simulink model "simulation"  (R2018b)
settings: Solver=ode45  StartTime=0.0  StopTime=36  FixedStep=0.00001  MaxStep=0.00001  MinStep=0.000005  RelTol=1e-3
settings Model: Creator=Dell  LastModifiedBy=Dell

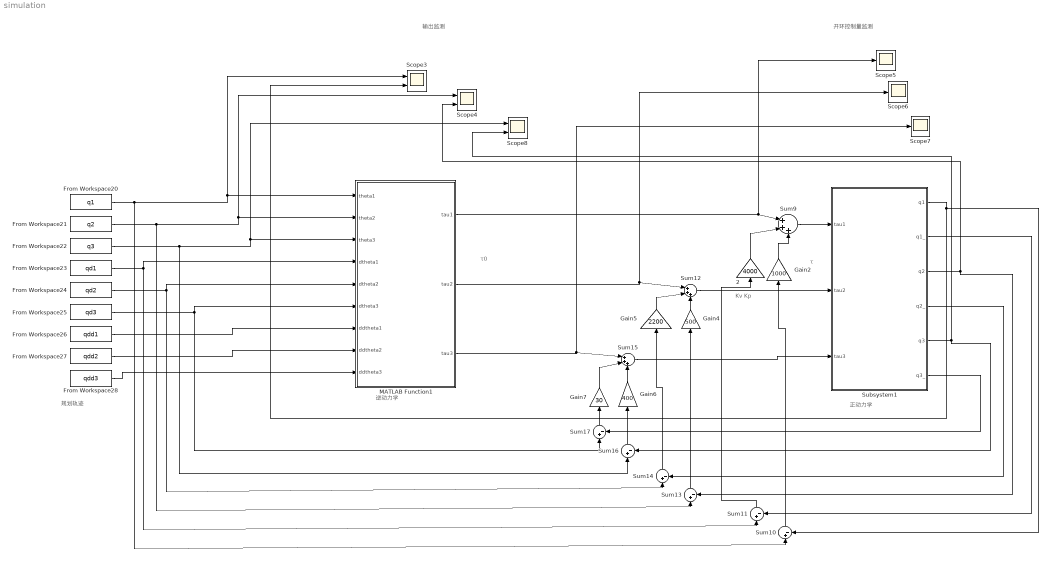
== system simulation ==
  note: 输出监测
  note: 正动力学
  note: 逆动力学
  note: 规划轨迹
  note: τ0
  note: Kv Kp
  note: τ
  note: 开环控制量监测
  2 : Gain  Gain=4000
  From Workspace20 : FromWorkspace  VariableName=q1  SampleTime=0
  From Workspace21 : FromWorkspace  VariableName=q2  SampleTime=0
  From Workspace22 : FromWorkspace  VariableName=q3  SampleTime=0
  From Workspace23 : FromWorkspace  VariableName=qd1  SampleTime=0
  From Workspace24 : FromWorkspace  VariableName=qd2  SampleTime=0
  From Workspace25 : FromWorkspace  VariableName=qd3  SampleTime=0
  From Workspace26 : FromWorkspace  VariableName=qdd1  SampleTime=0
  From Workspace27 : FromWorkspace  VariableName=qdd2  SampleTime=0
  From Workspace28 : FromWorkspace  VariableName=qdd3  SampleTime=0
  Gain2 : Gain  Gain=1000
  Gain4 : Gain  Gain=500
  Gain5 : Gain  Gain=2200
  Gain6 : Gain  Gain=400
  Gain7 : Gain  Gain=30
  MATLAB Function1 : MATLAB Function  TreatAsAtomicUnit=on
  Scope3 : Scope  NumInputPorts=2
  Scope4 : Scope  NumInputPorts=2
  Scope5 : Scope
  Scope6 : Scope
  Scope7 : Scope
  Scope8 : Scope  NumInputPorts=2
  Subsystem1 : Subsystem
  Sum{10..11,13..14,16..17} (6 alike) : Sum  Inputs=|+-
  Sum12 : Sum  Inputs=|+++
  Sum15 : Sum  Inputs=|+++
  Sum9 : Sum  Inputs=|+++
  wires:
  Subsystem1/1(q1) -> Scope3/2, Sum10/2
  From Workspace20/1 -> Scope3/1, MATLAB Function1/1(theta1), Sum10/1
  From Workspace25/1 -> Sum17/1, MATLAB Function1/6(dtheta3)
  From Workspace24/1 -> Sum14/1, MATLAB Function1/5(dtheta2)
  From Workspace28/1 -> MATLAB Function1/9(ddtheta3)
  From Workspace22/1 -> MATLAB Function1/3(theta3), Scope8/1, Sum16/1
  Subsystem1/5(q3) -> Sum16/2, Scope8/2
  From Workspace27/1 -> MATLAB Function1/8(ddtheta2)
  Subsystem1/3(q2) -> Sum13/2, Scope4/2
  From Workspace23/1 -> Sum11/1, MATLAB Function1/4(dtheta1)
  From Workspace26/1 -> MATLAB Function1/7(ddtheta1)
  MATLAB Function1/1(tau1) -> Scope5/1, Sum9/1
  Gain2/1 -> Sum9/3
  Sum10/1 -> Gain2/1
  Sum11/1 -> 2/1
  Subsystem1/2(q1_) -> Sum11/2
  2/1 -> Sum9/2
  Gain4/1 -> Sum12/3
  Gain5/1 -> Sum12/2
  MATLAB Function1/2(tau2) -> Scope6/1, Sum12/1
  Sum13/1 -> Gain4/1
  Sum14/1 -> Gain5/1
  Subsystem1/4(q2_) -> Sum14/2
  From Workspace21/1 -> Sum13/1, MATLAB Function1/2(theta2), Scope4/1
  Gain6/1 -> Sum15/3
  Gain7/1 -> Sum15/2
  MATLAB Function1/3(tau3) -> Scope7/1, Sum15/1
  Sum17/1 -> Gain7/1
  Sum16/1 -> Gain6/1
  Subsystem1/6(q3_) -> Sum17/2
  Sum9/1 -> Subsystem1/1(tau1)
  Sum12/1 -> Subsystem1/2(tau2)
  Sum15/1 -> Subsystem1/3(tau3)

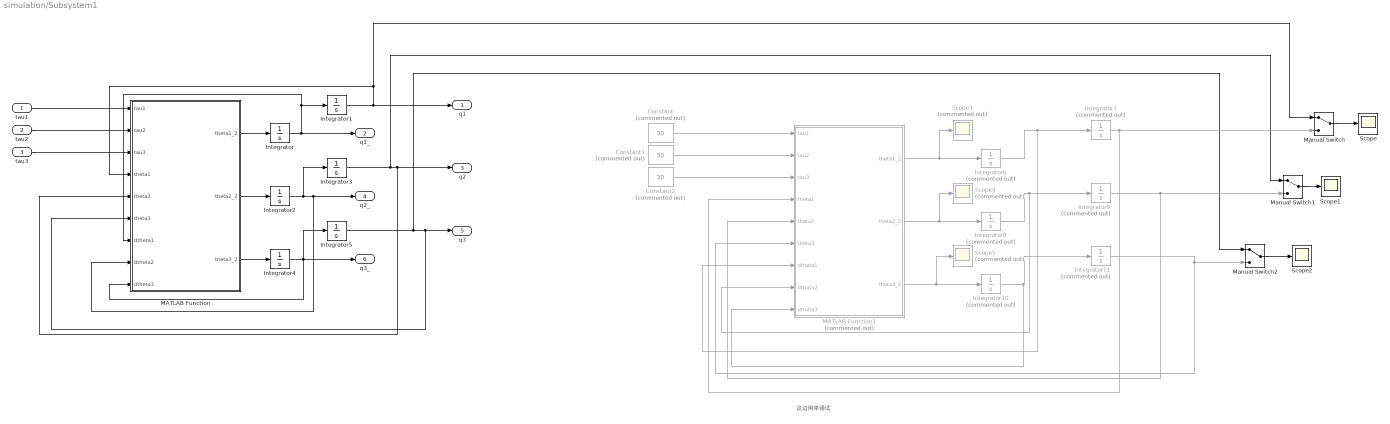
== system simulation/Subsystem1 ==
  note: 这边用来调试
  tau1 : Inport
  tau2 : Inport  Port=2
  tau3 : Inport  Port=3
  Constant : Constant  Commented=on  Value=30
  Constant1 : Constant  Commented=on  Value=30
  Constant2 : Constant  Commented=on  Value=30
  Integrator{,1..5} (6 alike) : Integrator  LimitOutput=on  UpperSaturationLimit=1000  LowerSaturationLimit=-1000
  Integrator{6..11} (6 alike) : Integrator  Commented=on
  MATLAB Function : MATLAB Function  TreatAsAtomicUnit=on
  MATLAB Function1 : MATLAB Function  Commented=on  TreatAsAtomicUnit=on
  Manual Switch : ManualSwitch
  Manual Switch1 : ManualSwitch
  Manual Switch2 : ManualSwitch
  Scope : Scope
  Scope1 : Scope
  Scope2 : Scope
  Scope3 : Scope  Commented=on
  Scope4 : Scope  Commented=on
  Scope5 : Scope  Commented=on
  q1 : Outport
  q1_ : Outport  Port=2
  q2 : Outport  Port=3
  q2_ : Outport  Port=4
  q3 : Outport  Port=5
  q3_ : Outport  Port=6
  wires:
  Integrator/1 -> MATLAB Function/7(dtheta1), Integrator1/1, q1_/1
  Integrator1/1 -> MATLAB Function/4(theta1), Manual Switch/1, q1/1
  Integrator2/1 -> MATLAB Function/8(dtheta2), q2_/1, Integrator3/1
  Integrator3/1 -> MATLAB Function/5(theta2), q2/1, Manual Switch1/1
  Integrator4/1 -> MATLAB Function/9(dtheta3), q3_/1, Integrator5/1
  Integrator5/1 -> Manual Switch2/1, MATLAB Function/6(theta3), q3/1
  tau1/1 -> MATLAB Function/1(tau1)
  tau2/1 -> MATLAB Function/2(tau2)
  tau3/1 -> MATLAB Function/3(tau3)
  MATLAB Function/1(theta1_2) -> Integrator/1
  MATLAB Function/2(theta2_2) -> Integrator2/1
  MATLAB Function/3(theta3_2) -> Integrator4/1
  Integrator9/1 -> Manual Switch1/2, MATLAB Function1/5(theta2)
  MATLAB Function1/3(theta3_2) -> Scope5/1, Integrator10/1
  Integrator11/1 -> Manual Switch2/2, MATLAB Function1/6(theta3)
  MATLAB Function1/2(theta2_2) -> Scope4/1, Integrator8/1
  Integrator7/1 -> Manual Switch/2, MATLAB Function1/4(theta1)
  MATLAB Function1/1(theta1_2) -> Integrator6/1, Scope3/1
  Constant/1 -> MATLAB Function1/1(tau1)
  Constant1/1 -> MATLAB Function1/2(tau2)
  Constant2/1 -> MATLAB Function1/3(tau3)
  Integrator6/1 -> Integrator7/1, MATLAB Function1/7(dtheta1)
  Integrator8/1 -> MATLAB Function1/8(dtheta2), Integrator9/1
  Integrator10/1 -> MATLAB Function1/9(dtheta3), Integrator11/1
  Manual Switch1/1 -> Scope1/1
  Manual Switch2/1 -> Scope2/1
  Manual Switch/1 -> Scope/1

== matlab function simulation/MATLAB Function1 ==
  data: theta1 input; tau1 output; theta2 input; theta3 input; dtheta1 input; dtheta2 input; dtheta3 input; ddtheta1 input; ddtheta2 input; ddtheta3 input; tau2 output; tau3 output
function [tau1,tau2,tau3] = fcu(theta1,theta2,theta3,dtheta1,dtheta2,dtheta3,ddtheta1,ddtheta2,ddtheta3)

    m1 = 10;
    m2 = 10;
    m3 = 10;
    L1 = 1;
    L2 = 1;
    L3 = 1;
    g = 10;
    
    A = [(L1^2*m1)/3 + L1^2*m2 + (L2^2*m2)/3 + (L3^2*m3)/12 + (m3*((L1 + L3/2 + L1*cos(theta2))*(2*L1 + L3 + 2*L1*cos(theta2)) + (L3 - 2*L1*sin(theta2))*(L3/2 - L1*sin(theta2))))/2 + L1*L2*m2 (L2^2*m2)/3 + (L3^2*m3)/12 + (m3*((L1 + L3/2)*(2*L1 + L3 + 2*L1*cos(theta2)) + (L3*(L3 - 2*L1*sin(theta2)))/2))/2 + (L1*L2*m2)/2 (L3^2*m3)/12 + (m3*((L3*(2*L1 + L3 + 2*L1*cos(theta2)))/2 + (L3*(L3 - 2*L1*sin(theta2)))/2))/2;
   (m3*(L3*(L3/2 - L1*sin(theta2)) + (2*L1 + L3)*(L1 + L3/2 + L1*cos(theta2))))/2 + (L2^2*m2)/3 + (L3^2*m3)/12 + (L1*L2*m2)/2 (m3*((2*L1 + L3)*(L1 + L3/2) + L3^2/2))/2 + (L2^2*m2)/3 + (L3^2*m3)/12 (m3*((L3*(2*L1 + L3))/2 + L3^2/2))/2 + (L3^2*m3)/12;
   (L3*m3*(6*L1 + 7*L3 + 6*L1*cos(theta2) - 6*L1*sin(theta2)))/12 (L3*m3*(6*L1 + 7*L3))/12 (7*L3^2*m3)/12
    ];

b=[(m3*(2*L1*dtheta2*sin(theta2)*((L3*(dtheta1 + dtheta2 + dtheta3))/2 + L1*(dtheta1 + dtheta2) + L1*dtheta1*cos(theta2)) + 2*L1*dtheta2*cos(theta2)*((L3*(dtheta1 + dtheta2 + dtheta3))/2 - L1*dtheta1*sin(theta2)) + L1*dtheta1*dtheta2*sin(theta2)*(2*L1 + L3 + 2*L1*cos(theta2)) + L1*dtheta1*dtheta2*cos(theta2)*(L3 - 2*L1*sin(theta2))))/2 - g*m3*(L2*cos(theta1 + theta2) + L1*cos(theta1) + (L3*cos(theta1 + theta2 + theta3))/2) - g*m2*((L2*cos(theta1 + theta2))/2 + L1*cos(theta1)) - (L1*g*m1*cos(theta1))/2
     (m3*(L1*L3*dtheta1*dtheta2*cos(theta2) + L1*dtheta1*dtheta2*sin(theta2)*(2*L1 + L3)))/2 - (m3*(2*L1*dtheta1*sin(theta2)*((L3*(dtheta1 + dtheta2 + dtheta3))/2 + L1*(dtheta1 + dtheta2) + L1*dtheta1*cos(theta2)) + 2*L1*dtheta1*cos(theta2)*((L3*(dtheta1 + dtheta2 + dtheta3))/2 - L1*dtheta1*sin(theta2))))/2 - g*m3*(L2*cos(theta1 + theta2) + (L3*cos(theta1 + theta2 + theta3))/2) - (L2*g*m2*cos(theta1 + theta2))/2
    (L3*m3*(6*L1*dtheta1*dtheta2*cos(theta2) - 6*g*cos(theta1 + theta2 + theta3) + 6*L1*dtheta1*dtheta2*sin(theta2)))/12];

    tau = A * [ddtheta1;ddtheta2;ddtheta3] - b;
    
    tau1 = tau(1);
    tau2 = tau(2);
    tau3 = tau(3);
    
end

== matlab function simulation/Subsystem1/MATLAB Function ==
  data: tau1 input; tau2 input; tau3 input; theta1_2 output; theta1 input; theta2 input; theta3 input; dtheta1 input; dtheta2 input; dtheta3 input; theta2_2 output; theta3_2 output
function [theta1_2 , theta2_2,theta3_2] = getTheta12(tau1,tau2,tau3,theta1,theta2,theta3,dtheta1,dtheta2,dtheta3)
    
    m1 = 10;
    m2 = 10;
    m3 = 10;
    L1 = 1;
    L2 = 1;
    L3 = 1;
    g = 10;

A=[(L1^2*m1)/3 + L1^2*m2 + (L2^2*m2)/3 + (L3^2*m3)/12 + (m3*((L1 + L3/2 + L1*cos(theta2))*(2*L1 + L3 + 2*L1*cos(theta2)) + (L3 - 2*L1*sin(theta2))*(L3/2 - L1*sin(theta2))))/2 + L1*L2*m2 (L2^2*m2)/3 + (L3^2*m3)/12 + (m3*((L1 + L3/2)*(2*L1 + L3 + 2*L1*cos(theta2)) + (L3*(L3 - 2*L1*sin(theta2)))/2))/2 + (L1*L2*m2)/2 (L3^2*m3)/12 + (m3*((L3*(2*L1 + L3 + 2*L1*cos(theta2)))/2 + (L3*(L3 - 2*L1*sin(theta2)))/2))/2;
   (m3*(L3*(L3/2 - L1*sin(theta2)) + (2*L1 + L3)*(L1 + L3/2 + L1*cos(theta2))))/2 + (L2^2*m2)/3 + (L3^2*m3)/12 + (L1*L2*m2)/2 (m3*((2*L1 + L3)*(L1 + L3/2) + L3^2/2))/2 + (L2^2*m2)/3 + (L3^2*m3)/12 (m3*((L3*(2*L1 + L3))/2 + L3^2/2))/2 + (L3^2*m3)/12;
   (L3*m3*(6*L1 + 7*L3 + 6*L1*cos(theta2) - 6*L1*sin(theta2)))/12 (L3*m3*(6*L1 + 7*L3))/12 (7*L3^2*m3)/12
    ];
b=[tau1 + (m3*(2*L1*dtheta2*sin(theta2)*((L3*(dtheta1 + dtheta2 + dtheta3))/2 + L1*(dtheta1 + dtheta2) + L1*dtheta1*cos(theta2)) + 2*L1*dtheta2*cos(theta2)*((L3*(dtheta1 + dtheta2 + dtheta3))/2 - L1*dtheta1*sin(theta2)) + L1*dtheta1*dtheta2*sin(theta2)*(2*L1 + L3 + 2*L1*cos(theta2)) + L1*dtheta1*dtheta2*cos(theta2)*(L3 - 2*L1*sin(theta2))))/2 - g*m3*(L2*cos(theta1 + theta2) + L1*cos(theta1) + (L3*cos(theta1 + theta2 + theta3))/2) - g*m2*((L2*cos(theta1 + theta2))/2 + L1*cos(theta1)) - (L1*g*m1*cos(theta1))/2
    tau2 + (m3*(L1*L3*dtheta1*dtheta2*cos(theta2) + L1*dtheta1*dtheta2*sin(theta2)*(2*L1 + L3)))/2 - (m3*(2*L1*dtheta1*sin(theta2)*((L3*(dtheta1 + dtheta2 + dtheta3))/2 + L1*(dtheta1 + dtheta2) + L1*dtheta1*cos(theta2)) + 2*L1*dtheta1*cos(theta2)*((L3*(dtheta1 + dtheta2 + dtheta3))/2 - L1*dtheta1*sin(theta2))))/2 - g*m3*(L2*cos(theta1 + theta2) + (L3*cos(theta1 + theta2 + theta3))/2) - (L2*g*m2*cos(theta1 + theta2))/2
    tau3 + (L3*m3*(6*L1*dtheta1*dtheta2*cos(theta2) - 6*g*cos(theta1 + theta2 + theta3) + 6*L1*dtheta1*dtheta2*sin(theta2)))/12];

theta_2 = b \ A;

theta1_2 = theta_2(1);
theta2_2 = theta_2(2);
theta3_2 = theta_2(3);

== matlab function simulation/Subsystem1/MATLAB Function1 ==
  data: tau1 input; tau2 input; tau3 input; theta1_2 output; theta1 input; theta2 input; theta3 input; dtheta1 input; dtheta2 input; dtheta3 input; theta2_2 output; theta3_2 output
function [theta1_2 , theta2_2,theta3_2] = getTheta12(tau1,tau2,tau3,theta1,theta2,theta3,dtheta1,dtheta2,dtheta3)
    
    m1 = 10;
    m2 = 10;
    m3 = 10;
    L1 = 1;
    L2 = 1;
    L3 = 1;
    g = 10;

A=[(L1^2*m1)/3 + L1^2*m2 + (L2^2*m2)/3 + (L3^2*m3)/12 + (m3*((L1 + L3/2 + L1*cos(theta2))*(2*L1 + L3 + 2*L1*cos(theta2)) + (L3 - 2*L1*sin(theta2))*(L3/2 - L1*sin(theta2))))/2 + L1*L2*m2 (L2^2*m2)/3 + (L3^2*m3)/12 + (m3*((L1 + L3/2)*(2*L1 + L3 + 2*L1*cos(theta2)) + (L3*(L3 - 2*L1*sin(theta2)))/2))/2 + (L1*L2*m2)/2 (L3^2*m3)/12 + (m3*((L3*(2*L1 + L3 + 2*L1*cos(theta2)))/2 + (L3*(L3 - 2*L1*sin(theta2)))/2))/2;
   (m3*(L3*(L3/2 - L1*sin(theta2)) + (2*L1 + L3)*(L1 + L3/2 + L1*cos(theta2))))/2 + (L2^2*m2)/3 + (L3^2*m3)/12 + (L1*L2*m2)/2 (m3*((2*L1 + L3)*(L1 + L3/2) + L3^2/2))/2 + (L2^2*m2)/3 + (L3^2*m3)/12 (m3*((L3*(2*L1 + L3))/2 + L3^2/2))/2 + (L3^2*m3)/12;
   (L3*m3*(6*L1 + 7*L3 + 6*L1*cos(theta2) - 6*L1*sin(theta2)))/12 (L3*m3*(6*L1 + 7*L3))/12 (7*L3^2*m3)/12
    ];
b=[tau1 + (m3*(2*L1*dtheta2*sin(theta2)*((L3*(dtheta1 + dtheta2 + dtheta3))/2 + L1*(dtheta1 + dtheta2) + L1*dtheta1*cos(theta2)) + 2*L1*dtheta2*cos(theta2)*((L3*(dtheta1 + dtheta2 + dtheta3))/2 - L1*dtheta1*sin(theta2)) + L1*dtheta1*dtheta2*sin(theta2)*(2*L1 + L3 + 2*L1*cos(theta2)) + L1*dtheta1*dtheta2*cos(theta2)*(L3 - 2*L1*sin(theta2))))/2 - g*m3*(L2*cos(theta1 + theta2) + L1*cos(theta1) + (L3*cos(theta1 + theta2 + theta3))/2) - g*m2*((L2*cos(theta1 + theta2))/2 + L1*cos(theta1)) - (L1*g*m1*cos(theta1))/2
    tau2 + (m3*(L1*L3*dtheta1*dtheta2*cos(theta2) + L1*dtheta1*dtheta2*sin(theta2)*(2*L1 + L3)))/2 - (m3*(2*L1*dtheta1*sin(theta2)*((L3*(dtheta1 + dtheta2 + dtheta3))/2 + L1*(dtheta1 + dtheta2) + L1*dtheta1*cos(theta2)) + 2*L1*dtheta1*cos(theta2)*((L3*(dtheta1 + dtheta2 + dtheta3))/2 - L1*dtheta1*sin(theta2))))/2 - g*m3*(L2*cos(theta1 + theta2) + (L3*cos(theta1 + theta2 + theta3))/2) - (L2*g*m2*cos(theta1 + theta2))/2
    tau3 + (L3*m3*(6*L1*dtheta1*dtheta2*cos(theta2) - 6*g*cos(theta1 + theta2 + theta3) + 6*L1*dtheta1*dtheta2*sin(theta2)))/12];

theta_2 = inv(A) * b;

theta1_2 = theta_2(1);
theta2_2 = theta_2(2);
theta3_2 = theta_2(3);
